simulink model "Open_Loop_Simulation"  (R2018b)
settings: Solver=FixedStepDiscrete  StartTime=0.0  StopTime=inf  FixedStep=0.01  RelTol=1e-3
settings Model: EnablePacing=on  PacingRate=2  Creator=Daniele Nava  LastModifiedBy=Daniele Nava

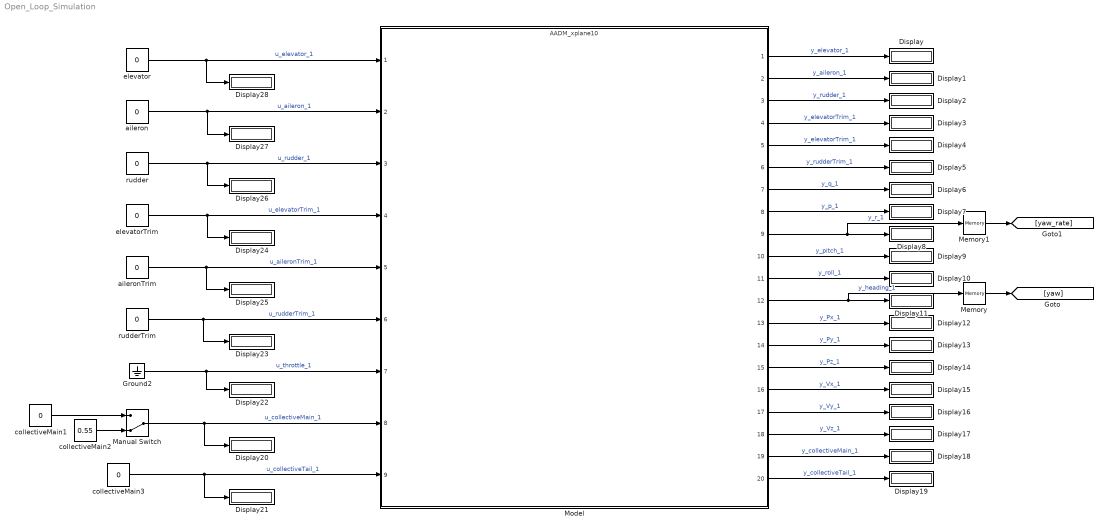
== system Open_Loop_Simulation ==
  Display{,1..28} (29 alike) : Display
  Ground2 : Ground
  Manual Switch : ManualSwitch  CurrentSetting=0
  Memory : Memory
  Memory1 : Memory
  Model : ModelReference  ModelNameDialog=AADM_xplane10.slx  SimulationMode=Normal  ModelReferenceVersion=1.10
  aileron : Constant  Value=0
  aileronTrim : Constant  Value=0
  collectiveMain1 : Constant  Value=0
  collectiveMain2 : Constant  Value=0.55
  collectiveMain3 : Constant  Value=0
  elevator : Constant  Value=0
  elevatorTrim : Constant  Value=0
  rudder : Constant  Value=0
  rudderTrim : Constant  Value=0
  wires:
  elevatorTrim/1 -> Display24/1, Model/4  "u_elevatorTrim_1"
  elevator/1 -> Display28/1, Model/1  "u_elevator_1"
  aileron/1 -> Display27/1, Model/2  "u_aileron_1"
  aileronTrim/1 -> Display25/1, Model/5  "u_aileronTrim_1"
  rudderTrim/1 -> Display23/1, Model/6  "u_rudderTrim_1"
  Model/2 -> Display1/1  "y_aileron_1"
  Model/9 -> Memory1/1, Display8/1  "y_r_1"
  Model/17 -> Display16/1  "y_Vy_1"
  Model/18 -> Display17/1  "y_Vz_1"
  Model/19 -> Display18/1  "y_collectiveMain_1"
  Model/10 -> Display9/1  "y_pitch_1"
  Model/13 -> Display12/1  "y_Px_1"
  Model/14 -> Display13/1  "y_Py_1"
  Model/12 -> Memory/1, Display11/1  "y_heading_1"
  Model/4 -> Display3/1  "y_elevatorTrim_1"
  Model/5 -> Display4/1  "y_elevatorTrim_1"
  Model/20 -> Display19/1  "y_collectiveTail_1"
  Model/8 -> Display7/1  "y_p_1"
  Model/7 -> Display6/1  "y_q_1"
  Model/16 -> Display15/1  "y_Vx_1"
  Model/15 -> Display14/1  "y_Pz_1"
  Model/1 -> Display/1  "y_elevator_1"
  Model/11 -> Display10/1  "y_roll_1"
  Model/3 -> Display2/1  "y_rudder_1"
  Model/6 -> Display5/1  "y_rudderTrim_1"
  Ground2/1 -> Display22/1, Model/7  "u_throttle_1"
  Memory/1 -> [yaw]
  Manual Switch/1 -> Display20/1, Model/8  "u_collectiveMain_1"
  collectiveMain3/1 -> Display21/1, Model/9  "u_collectiveTail_1"
  rudder/1 -> Display26/1, Model/3  "u_rudder_1"
  collectiveMain1/1 -> Manual Switch/1
  collectiveMain2/1 -> Manual Switch/2
  Memory1/1 -> [yaw_rate]
